simulink model "zad2_wariant2"  (R2017a)
settings: Solver=VariableStepAuto  StartTime=0.0  StopTime=400  RelTol=1e-3
values from neighbouring files (symbols this model uses):
  Tp = 0.1    [zad3a.m]    (also in zad3b.m; zad3max.m; zad4.m)
settings Model: Creator=Rajtek  LastModifiedBy=Rajtek

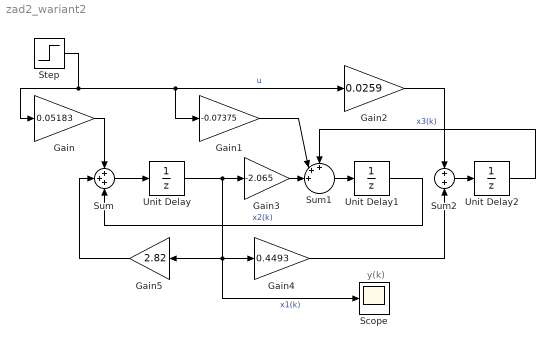
== system zad2_wariant2 ==
  note: y(k)
  Gain : Gain  Gain=0.05183
  Gain1 : Gain  Gain=-0.07375
  Gain2 : Gain  Gain=0.0259
  Gain3 : Gain  Gain=-2.065
  Gain4 : Gain  Gain=0.4493
  Gain5 : Gain  Gain=2.82
  Scope : Scope
  Step : Step  SampleTime=0
  Sum : Sum  Inputs=+++
  Sum1 : Sum  Inputs=+++||
  Sum2 : Sum  Inputs=+|+
  Unit Delay : UnitDelay  SampleTime=Tp
  Unit Delay1 : UnitDelay  SampleTime=Tp
  Unit Delay2 : UnitDelay  SampleTime=Tp
  wires:
  Sum2/1 -> Unit Delay2/1
  Sum1/1 -> Unit Delay1/1
  Unit Delay/1 -> Scope/1, Gain4/1, Gain5/1, Gain3/1  "x1(k)"
  Gain/1 -> Sum/1
  Step/1 -> Gain/1, Gain2/1, Gain1/1  "u"
  Sum/1 -> Unit Delay/1
  Gain2/1 -> Sum2/1
  Gain1/1 -> Sum1/2
  Gain5/1 -> Sum/2
  Gain4/1 -> Sum2/2
  Unit Delay2/1 -> Sum1/1  "x3(k)"
  Gain3/1 -> Sum1/3
  Unit Delay1/1 -> Sum/3  "x2(k)"
